simulink model "power_kundur_statcom01"  (R2021a)
settings: Solver=ode23tb  StartTime=0.0  StopTime=10  MaxStep=1/60  RelTol=1e-4  EnableMultiTasking=on
values from neighbouring files (symbols this model uses):
  j = 1    [OABC_PSO_TUNED_NOFault.mat]    (also in OABC_PSO_TUNED_ThreePHASEFault.mat; Traditional_ABC_PSO2.m = randi([1 noFood], 1))
  kk = [0 0.302628193662]    [OABC_PSO_TUNED_NOFault.mat]    (also in OABC_PSO_TUNED_ThreePHASEFault.mat = [6.69502367045 1584.585174])
undefined symbols (not defined in the file or in its folder): Ac, Bc, Cc, D1, Dc, Delta, Fnom, gcbh, K_Vdq2m_SH, Kf_I_SH, Ki_I_SH, Ki_Vac_SH, Ki_Vdc_SH, Kp_I_SH, Kp_Vac_SH, Kp_Vdc_SH, L_RL_SH, MagIinit_SH, PhaIinit_SH, R_RL_SH, sps_rtmsupport, VdcRef_SH, Vnom_SH, xfo_ratio_SH
libraries: spsGenericPowerSystemStabilizerLib x8, spsLoadFlowBusLib x6, spsThreePhaseParallelRLCLoadLib x4, spsThreePhasePISectionLineLib x4, spsSynchronousMachinepuStandardLib x4, spsExcitationSystemLib x4, spsMultiBandPowerSystemStabilizerLib x4, spsSteamTurbineandGovernorLib x4, spsThreePhaseTransformerTwoWindingsLib x4, spsThreePhaseVIMeasurementLib x3, spsThreePhaseBreakerLib x2, spsControlledCurrentSourceLib x2
(part 1 of 3)
Description:
  | Copyright 2008-2015 The MathWorks, Inc.
settings Model: FPTRunName=Active  ExtModeTrigMode=oneshot  ExtModeArmWhenConnect=off  ExtModeAutoUpdateStatusClock=off  Creator=MathWorks  LastModifiedBy=USER
settings SolverCC: AlgebraicLoopSolver=TrustRegion
settings DataIOCC: SaveFormat=Array  SignalLoggingSaveFormat=ModelDataLogs  SaveOutput=off  SaveTime=off  ReturnWorkspaceOutputs=off  TimeSaveName=t  SignalLoggingName=sigsOut
settings OptimizationCC: BlockReduction=off  BooleanDataType=off  ExpressionDepthLimit=2147483647  InitFltsAndDblsToZero=on  LifeSpan=inf
settings DebuggingCC: UnderspecifiedInitializationDetection=Classic  MergeDetectMultiDrivingBlocksExec=none  SignalResolutionControl=TryResolveAllWithWarning  MultiTaskDSMMsg=warning  MultiTaskCondExecSysMsg=none  FcnCallInpInsideContextMsg=warning  UnconnectedOutputMsg=none  StateNameClashWarn=warning  SFUnexpectedBacktrackingDiag=warning  SFNoUnconditionalDefaultTransitionDiag=warning  SFExecutionAtInitializationDiag=none  SFMachineParentedDataDiag=warning  ArithmeticOperatorsInVariantConditions=warning
settings HardwareCC: ProdBitPerPointer=32  ProdBitPerSizeT=32  ProdBitPerPtrDiffT=32  ProdLargestAtomicFloat=None  ProdIntDivRoundTo=Undefined  ProdEndianess=Unspecified  ProdWordSize=32  ProdHWDeviceType=32-bit Generic  TargetUnknown=on
settings ModelReferenceCC: PropagateSignalLabelsOutOfModel=off
settings SFSimCC: SimUseLocalCustomCode=off  CustomCodeUndefinedFunction=UseInterfaceOnly
settings RTWCC: RTWUseLocalCustomCode=off
settings CodeAppCC: StateflowObjectComments=on
settings GRTTargetCC: TargetLangStandard=C89/C90 (ANSI)  CombineOutputUpdateFcns=off  GRTInterface=on
settings ConfigComp: CovMetricSettings=dw  CovSaveCumulativeToWorkspaceVar=on  CovSaveSingleToWorkspaceVar=on  CovExternalEMLEnable=off  CovSFcnEnable=off
settings SimscapeCC: SimscapeNormalizeSystem=off

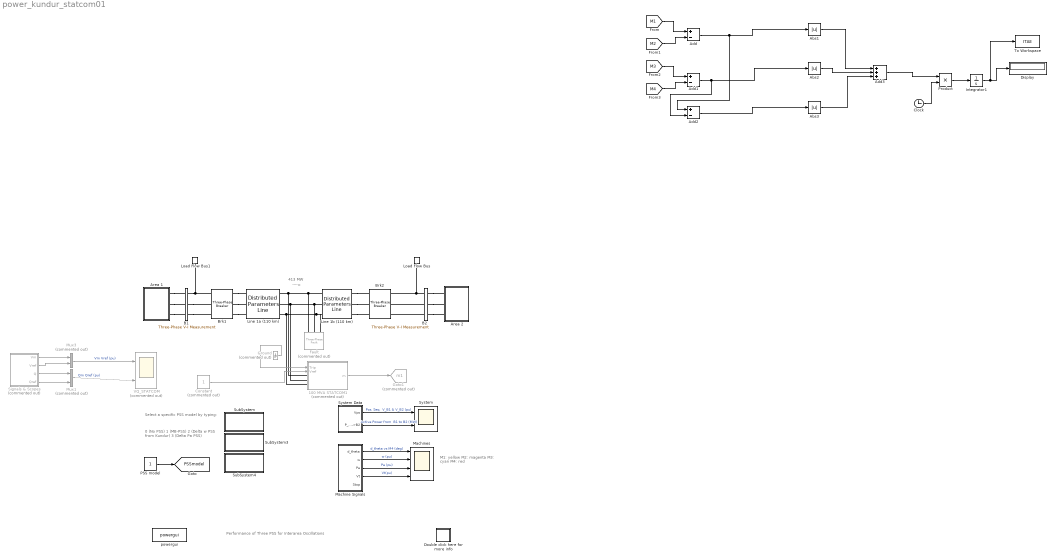
== system power_kundur_statcom01 ==
  note: Performance of Three PSS for Interarea Oscillations
  note: M1: yellow
      | M2: magenta
      | M3: cyan
      | M4: red
  note: ---->
  note: 413 MW
  note: Select a specific PSS model
      | by typing:
  note: 0  (No PSS)
      | 1  (MB-PSS)
      | 2  (Delta w PSS from Kundur)
      | 3  (Delta Pa PSS)
  " Brk2" : spsThreePhaseBreakerLib/Three-Phase Breaker  InitialState=closed  SwitchA=off  SwitchB=off  SwitchC=off  SwitchTimes=[1+8/60]  External=off  BreakerResistance=0.001  SnubberResistance=1e6  SnubberCapacitance=0  Measurements=None
      settings: AttributesFormatString=\n
  100 MVA STATCOM1 : Subsystem  Commented=on  AncestorBlock=|  DialogController=POWERSYS.PowerSysDialog  LoadFcn=sps_rtmsupport('LoadFcn',gcbh);  StartFcn=sps_rtmsupport('StartFcn',gcbh);  StopFcn=sps_rtmsupport('StopFcn',gcbh);  mask(Static Synchronous Compensator (Phasor Type)){SystemNominal=[ 230e3, 60 ], Pnom_SH=200e6, RL_SH=[ 0.071, 0.22 ], Iinit_SH=[0, 0 ], VnomDC=40000, C_DC=750e-6/2, OpMode_SH=Voltage regulation, Vref_SH=1.00, ExternalVref=on, MaxRateChangeVref_SH=100, Droop_SH=0.03, Par_VacReg=[kk(1) kk(2)], Qref_SH=0, MaxRateChangeQref_SH=2, Par_VdcReg=[kk(3) kk(4)], Par_IReg_SH=[0.3 10 0.22]}
      | factslib/Power-Electronics Based
      | FACTS/Static Synchronous
      | Compensator
      | (Phasor Type)
      mask prompts: SystemNominal "Nominal voltage and frequency [Vrms L-L, fn(Hz)]:"; Pnom_SH "Converter rating (VA):"; RL_SH "Converter impedance [R(pu), L(pu)]:"; Iinit_SH "Converter initial current [Mag(pu), Pha(deg.)]:"; VnomDC "DC link nominal voltage (V):"; C_DC "DC link total equivalent capacitance (F):"; OpMode_SH "Mode:"; Vref_SH "Reference voltage Vref (pu):"; ExternalVref "External"; MaxRateChangeVref_SH "Maximum rate of change of reference voltage (pu/s):"; Droop_SH "Droop (pu):"; Par_VacReg "Vac Regulator gains [Kp, Ki]:"; Qref_SH "Reactive power setpoint Qref (pu):"; MaxRateChangeQref_SH "Maximum rate of change of reactive power setpoint (pu/s):"; Par_VdcReg "Vdc Regulator gains [Kp, Ki]:"; Par_IReg_SH "Current Regulator gains [Kp, Ki, Kf];"
      mask help: Implement phasor model of three-phase static synchronous compensator (STATCOM).
      mask init:
      | [ j,Fnom,Vnom_SH,VdcRef_SH,R_RL_SH,L_RL_SH,Kp_Vac_SH,Ki_Vac_SH,Kp_Vdc_SH,Ki_Vdc_SH,Kp_I_SH,Ki_I_SH,Kf_I_SH,VconvMax_pu,VconvMaxPrim,m_max,VconvMaxSec,xfo_ratio_SH,K_Vdq2m_SH,a,a2,MagIinit_SH,PhaIinit_SH] = powericon('StatcomInit',SystemNominal,VnomDC,Par_VacReg, Par_VdcReg, Par_IReg_SH,Iinit_SH,gcbh,RL_SH);
      settings: CopyFcn=sps_rtmsupport('CopyFcn',gcbh);  DeleteFcn=sps_rtmsupport('DeleteFcn',gcbh);  UndoDeleteFcn=sps_rtmsupport('UndoDeleteFcn',gcbh);  ModelCloseFcn=sps_rtmsupport('ModelCloseFcn',gcbh);  PreSaveFcn=sps_rtmsupport('PreSaveFcn',gcbh);  PostSaveFcn=sps_rtmsupport('PostSaveFcn',gcbh);  NameChangeFcn=sps_rtmsupport('NameChangeFcn',gcbh);  PreCopyFcn=sps_rtmsupport('PreCopyFcn',gcbh);  OpenFcn=sps_rtmsupport('OpenFcn',gcbh, [7 9]);  CloseFcn=sps_rtmsupport('CloseFcn',gcbh);  PreDeleteFcn=sps_rtmsupport('PreDeleteFcn',gcbh);
      mask Help: helpview(psbhelp);
      mask TypeOptions OpMode_SH: Var Control | Voltage regulation
      mask Callback OpMode_SH: StatcomCback(gcbh);
      mask Callback ExternalVref: StatcomCback(gcbh);
      mask DialogControl powerdata Prompt: Power
      mask DialogControl control Prompt: Controller
      mask Display:
      | color('blue');
      | disp('STATCOM')
  Abs1 : Abs
  Abs2 : Abs
  Abs3 : Abs
  Add : Sum  Inputs=+-
  Add1 : Sum  Inputs=+-
  Add2 : Sum  Inputs=+-
  Add3 : Sum  Inputs=+++
  Area 1 : Subsystem
  Area 2 : Subsystem
  B1 : spsThreePhaseVIMeasurementLib/Three-Phase V-I Measurement  VoltageMeasurement=phase-to-ground  SetLabelV=on  LabelV=Vabc_B1  Vpu=off  VpuLL=off  CurrentMeasurement=yes  SetLabelI=on  LabelI=Iabc_B1  Ipu=off  Pbase=100e6  Vbase=500e3  OutputType=Complex  PhasorSimulation=on  PSBequivalent=0
  B2 : spsThreePhaseVIMeasurementLib/Three-Phase V-I Measurement  VoltageMeasurement=phase-to-ground  SetLabelV=on  LabelV=Vabc_B2  Vpu=off  VpuLL=off  CurrentMeasurement=yes  SetLabelI=on  LabelI=Iabc_B2  Ipu=off  Pbase=100e6  Vbase=500e3  OutputType=Complex  PhasorSimulation=on  PSBequivalent=0
  Brk1 : spsThreePhaseBreakerLib/Three-Phase Breaker  InitialState=closed  SwitchA=off  SwitchB=off  SwitchC=off  SwitchTimes=[1+8/60]  External=off  BreakerResistance=0.001  SnubberResistance=inf  SnubberCapacitance=0  Measurements=None
      settings: AttributesFormatString=\n
  Clock : Clock
  Constant : Constant  Commented=on
  Display : Display
  Double click here for more info : Subsystem
      settings: OpenFcn=showdemo(bdroot(gcb))
      mask Display: disp('?')
  Fault : spsThreePhaseFaultLib/Three-Phase Fault  Commented=on  InitialStates=0  FaultA=on  FaultB=on  FaultC=on  GroundFault=on  SwitchTimes=[ 1 1+12/60]  External=off  SwitchStatus=NaN  FaultResistance=0.001  GroundResistance=0.001  SnubberResistance=inf  SnubberCapacitance=0  Measurements=Fault voltages and currents
  Goto1 : Goto  Commented=on  GotoTag=m1  TagVisibility=global
  Ground : Ground  Commented=on
  Integrator1 : Integrator
  Line 1a (110 km) : spsDistributedParametersLineLib/Distributed Parameters Line  Phases=3  Length=110  Frequency=60  Resistance=[0.0001*529 1.61]  Inductance=[0.001*529/(377) 0.0061]  Capacitance=[0.00175/529/(377) 5.2489e-9]  x1=[1.07105753768753e-08 249286.617062631 249286.103987125;376.991118430775 376.991118430775 376.991118430775;-0.430181636815253 0.685365733894338 -0.885427065915489]  x2=[1.12823805694267e-08 223892.22603189 223891.788922386;376.991118430775 376.991118430775 376.991118430775;-0.654447081019999 0.431460957299027 -1.13933225811238]  x3=[6.57239902882849e-12 568.631458690706 568.631298110426;376.991118430775 376.991118430775 376.991118430775;-1.56783526225894 3.01615797225432 1.44536743576562]  x4=[1.40882222020251e-11 1660.67806578935 1660.67616695075;376.991118430775 376.991118430775 376.991118430775;-0.32396524232274 0.29261475856702 -1.27817771618835]  x5=0.000622431770558027  V1=ones(3,3)  V2=ones(3,3)  I1=ones(3,3)  I2=ones(3,3)  nHarmo=1  Measurements=None  Decoupling=off  VsMag0=0  VrMag0=0  VsAngle0=0  VrAngle0=0  IsMag0=0  IrMag0=0  IsAngle0=0  IrAngle0=0
      settings: AttributesFormatString=\n  SourceProductBaseCode=PS
  Line 1b (110 km) : spsDistributedParametersLineLib/Distributed Parameters Line  Phases=3  Length=110  Frequency=60  Resistance=[0.0001*529 1.61]  Inductance=[0.001*529/(377) 0.0061]  Capacitance=[0.00175/529/(377) 5.2489e-9]  x1=[1.12823805694267e-08 223892.22603189 223891.788922386;376.991118430775 376.991118430775 376.991118430775;-0.654447081019999 0.431460957299027 -1.13933225811238]  x2=[1.2011449678639e-08 211111.793515844 211111.458207578;376.991118430775 376.991118430775 376.991118430775;-0.792576364184504 0.132665789252052 -1.4381277782236]  x3=[8.25606215961616e-12 584.178043584259 584.177876576689;376.991118430775 376.991118430775 376.991118430775;-1.38577443880165 -3.11450148556165 1.59789324135678]  x4=[1.24190041898095e-11 1644.49352968555 1644.49164426305;376.991118430775 376.991118430775 376.991118430775;-0.543069260432015 0.147593243960904 -1.42319923514757]  x5=0.000622431770558027  V1=ones(3,3)  V2=ones(3,3)  I1=ones(3,3)  I2=ones(3,3)  nHarmo=1  Measurements=None  Decoupling=off  VsMag0=0  VrMag0=0  VsAngle0=0  VrAngle0=0  IsMag0=0  IrMag0=0  IsAngle0=0  IrAngle0=0
      settings: AttributesFormatString=\n  SourceProductBaseCode=PS
  Load Flow Bus : spsLoadFlowBusLib/Load Flow Bus  LConnTagsString=a  Phases=single  Connectors=on one side  ID=B2  Vbase=230e3  Vref=1  Vangle=0  VLF=1.003  VLFb=1  VLFc=1  angleLF=-11.43  angleLFb=0  angleLFc=0
      settings: AttributesFormatString=%<ID>\n%<Vbase>V\n%<VLF>pu\n%<angleLF>deg.  SourceProductBaseCode=PS
  Load Flow Bus1 : spsLoadFlowBusLib/Load Flow Bus  LConnTagsString=a  Phases=single  Connectors=on one side  ID=B1  Vbase=230e3  Vref=1  Vangle=0  VLF=0.9916  VLFb=1  VLFc=1  angleLF=15.06  angleLFb=0  angleLFc=0
      settings: AttributesFormatString=%<ID>\n%<Vbase>V\n%<VLF>pu\n%<angleLF>deg.  SourceProductBaseCode=PS
  Machine Signals : Subsystem
  Machines : Scope  NumInputPorts=4
  Mux1 : Mux  Commented=on  Inputs=2
  Mux3 : Mux  Commented=on  Inputs=2
  PSS model : Constant
  Product : Product
  Signals & Scopes : Subsystem  Commented=on
  SubSystem : Subsystem
      settings: OpenFcn=openfig('psbPSSbode.fig');
      mask Display: disp('Show Bode plot \nof PSS')
  SubSystem3 : Subsystem
      settings: OpenFcn=openfig('psbPSSstep.fig');
      mask Display: disp('Show results: \nStep on vref\nof M1')
  SubSystem4 : Subsystem
      settings: OpenFcn=openfig('psbPSSfault.fig');
      mask Display: disp('Show results: \n3-phase fault')
  System : Scope  NumInputPorts=2
  System Data : Subsystem
  To Workspace : ToWorkspace  VariableName=ITAE  SampleTime=-1
      settings: Save2DSignal=2-D array (concatenate along first dimension)
  VQ_STATCOM : Scope  Commented=on  NumInputPorts=2
  powergui : spspowerguiLib/powergui  Priority=2  SimulationMode=Phasor  SampleTime=0  frequency=60  Iterations=50  frequencyindice=60  Pbase=100e6  ErrMax=0.0001  UnitsV=kV  UnitsW=MW  buscounter=0  FunctionMessages=off  echomessages=on  EnableUseOfTLC=off  CurrentSourceSwitches=off  DisableSnubberDevices=off  DisableRonSwitches=off  DisableVfSwitches=off  DisplayEquations=off  AutomaticDiscreteSolvers=off  SolverType=Tustin  Interpol=off  ExternalGateDelay=off  methode=off  Ts=0  x0status=blocks  SPID=off  SwTol=0  HookPort=off  NonlinearTolerance=1e-4  nMaxIteration=100  ContinueOnMaxIteration=off  RestoreLinks=warning  ResistiveCurrentMeasurement=off  Frange=logspace(0,3,50)  Ylog=off  Xlog=off  ShowGrid=off  save=off  variable=ZData  structure=0  ZoomFFT=on  StartTime=0.0  cycles=1  DisplayStyle=1  fundamental=60  FreqAxis=off  MaxFrequency=1000  frequencyindicesteady=1  RmsSteady=1  display=off
  tag scope: PSSmodel=global
  wires:
  Machine Signals/1(d_theta) -> Machines/1  "d_theta vs M4 (deg)"
  Machine Signals/2(w) -> Machines/2  "w (pu)"
  Machine Signals/3(Pa) -> Machines/3  "Pa (pu)"
  Machine Signals/4(Vt) -> Machines/4  "Vt(pu)"
  System Data/1(Vps) -> System/1  "Pos. Seq.  V_B1 & V_B2 (pu)"
  System Data/2(P_B1->B2) -> System/2  "Active Power from  B1 to B2 (MW)"
  PSS model/1 -> [PSSmodel]
  Constant/1 -> 100 MVA STATCOM1/2("Vref ")
  Ground/1 -> 100 MVA STATCOM1/1(Trip)
  Signals & Scopes/1(Vm) -> Mux3/1
  Signals & Scopes/2(Vref) -> Mux3/2
  Signals & Scopes/3(Q) -> Mux1/1
  Signals & Scopes/4(Qref) -> Mux1/2
  Mux3/1 -> VQ_STATCOM/1  "Vm Vref (pu)"
  Mux1/1 -> VQ_STATCOM/2  "Qm Qref (pu)"
  100 MVA STATCOM1/1(m) -> Goto1/1
  Clock/1 -> Product/2
  Product/1 -> Integrator1/1
  Integrator1/1 -> To Workspace/1, Display/1
  [M1] -> Add/1
  [M2] -> Add/2
  Add/1 -> Add2/1, Abs1/1
  Add1/1 -> Add2/2, Abs2/1
  [M3] -> Add1/1
  [M4] -> Add1/2
  Add2/1 -> Abs3/1
  Abs1/1 -> Add3/1
  Abs2/1 -> Add3/2
  Abs3/1 -> Add3/3
  Add3/1 -> Product/1
  connections:
  Brk1/RConn1 -- Line 1a (110 km)/LConn1
  Brk1/RConn2 -- Line 1a (110 km)/LConn2
  Brk1/RConn3 -- Line 1a (110 km)/LConn3
  Line 1b (110 km)/LConn1 -- 100 MVA STATCOM1/LConn1 -- Line 1a (110 km)/RConn1 -- Fault/LConn1
  Line 1b (110 km)/LConn2 -- 100 MVA STATCOM1/LConn2 -- Line 1a (110 km)/RConn2 -- Fault/LConn2
  Line 1a (110 km)/RConn3 -- Line 1b (110 km)/LConn3 -- Fault/LConn3 -- 100 MVA STATCOM1/LConn3
  Line 1b (110 km)/RConn1 -- " Brk2"/LConn1
  Line 1b (110 km)/RConn2 -- " Brk2"/LConn2
  Line 1b (110 km)/RConn3 -- " Brk2"/LConn3
  Area 1/RConn2 -- B1/LConn2
  Area 1/RConn1 -- B1/LConn1
  Area 1/RConn3 -- B1/LConn3
  B1/RConn2 -- Brk1/LConn2
  B1/RConn1 -- Brk1/LConn1 -- Load Flow Bus1/LConn1
  B1/RConn3 -- Brk1/LConn3
  B2/RConn2 -- Area 2/LConn2
  B2/RConn1 -- Area 2/LConn1
  B2/RConn3 -- Area 2/LConn3
  B2/LConn2 -- " Brk2"/RConn2
  B2/LConn1 -- " Brk2"/RConn1 -- Load Flow Bus/LConn1
  B2/LConn3 -- " Brk2"/RConn3

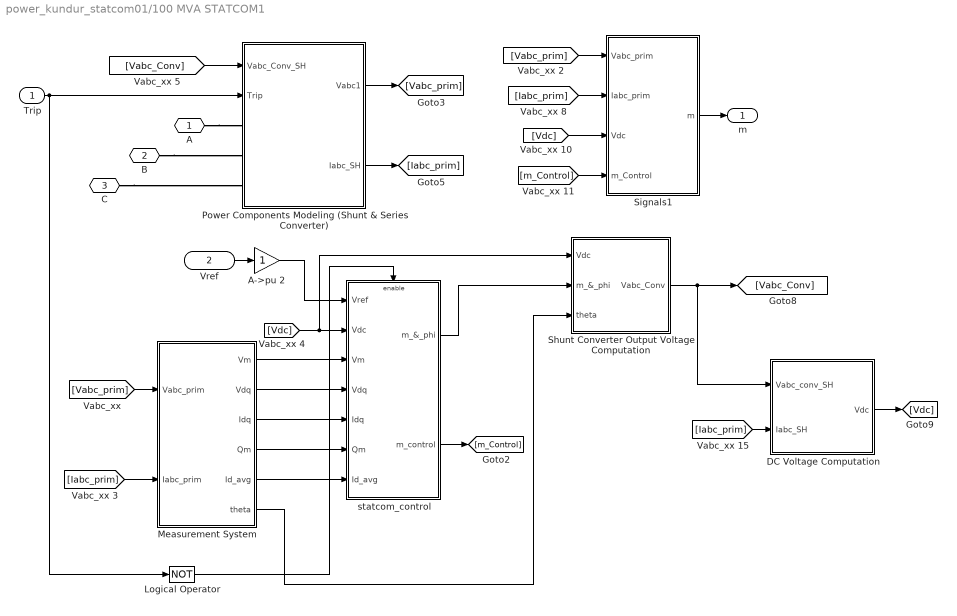
== system power_kundur_statcom01/100 MVA STATCOM1 ==
  Trip : Inport
  "Vref " : Inport  Port=2
  A->pu 2 : Gain  SaturateOnIntegerOverflow=on  SampleTime=0  OutDataTypeStr=Inherit: Same as input  ParamDataTypeStr=Inherit: Same as input
  DC Voltage Computation : Subsystem
  Logical Operator : Logic  Operator=NOT  AllPortsSameDT=off  OutDataTypeStr=float('double')  SampleTime=0
  Measurement System : Subsystem  mask{Vm_SH_Init=1, Id_avg_SH_Init=0, Qm_SH_Init=0, Fnom=Fnom, Vnom_SH=Vnom_SH, Pnom_SH=Pnom_SH}
      mask prompts: Vm_SH_Init "Initial value for Vm_SH (pu):"; Id_avg_SH_Init "Initial value for Id_avg_SH (pu):"; Qm_SH_Init "Initial value for Qm_SH (pu):"; Fnom "System frequency (Hz):"
  Power Components Modeling (Shunt & Series Converter) : Subsystem
  Shunt Converter Output Voltage Computation : Subsystem
  Signals1 : Subsystem
  statcom_control : Subsystem
  "A " : PMIOPort  Side=Left
  B : PMIOPort  Port=2  Side=Left
  C : PMIOPort  Port=3  Side=Left
  m : Outport  VectorParamsAs1DForOutWhenUnconnected=off
  wires:
  statcom_control/2(m_control) -> [m_Control]
  Logical Operator/1 -> statcom_control/Enable
  Measurement System/5(Id_avg) -> statcom_control/7(Id_avg)
  Measurement System/4(Qm) -> statcom_control/6(Qm)
  Trip/1 -> Logical Operator/1, Power Components Modeling (Shunt & Series Converter)/2(Trip)
  Measurement System/6(theta) -> Shunt Converter Output Voltage Computation/3(theta)
  [Vdc] -> statcom_control/2(Vdc), Shunt Converter Output Voltage Computation/1(Vdc)
  A->pu 2/1 -> statcom_control/1(Vref)
  [Vabc_prim] -> Measurement System/1(Vabc_prim)
  [Iabc_prim] -> Measurement System/2(Iabc_prim)
  Measurement System/3(Idq) -> statcom_control/5(Idq)
  Measurement System/2(Vdq) -> statcom_control/4(Vdq)
  Measurement System/1(Vm) -> statcom_control/3(Vm)
  DC Voltage Computation/1(Vdc) -> [Vdc]
  [Iabc_prim] -> DC Voltage Computation/2(Iabc_SH)
  Shunt Converter Output Voltage Computation/1(Vabc_Conv) -> DC Voltage Computation/1(Vabc_conv_SH), [Vabc_Conv]
  [m_Control] -> Signals1/4(m_Control)
  [Vdc] -> Signals1/3(Vdc)
  [Iabc_prim] -> Signals1/2(Iabc_prim)
  [Vabc_prim] -> Signals1/1(Vabc_prim)
  Power Components Modeling (Shunt & Series Converter)/2(Iabc_SH) -> [Iabc_prim]
  Power Components Modeling (Shunt & Series Converter)/1(Vabc1) -> [Vabc_prim]
  [Vabc_Conv] -> Power Components Modeling (Shunt & Series Converter)/1(Vabc_Conv_SH)
  Signals1/1(m) -> m/1
  statcom_control/1(m_&_phi) -> Shunt Converter Output Voltage Computation/2(m_&_phi)
  "Vref "/1 -> A->pu 2/1
  connections:
  C/RConn1 -- Power Components Modeling (Shunt & Series Converter)/LConn3
  B/RConn1 -- Power Components Modeling (Shunt & Series Converter)/LConn2
  "A "/RConn1 -- Power Components Modeling (Shunt & Series Converter)/LConn1

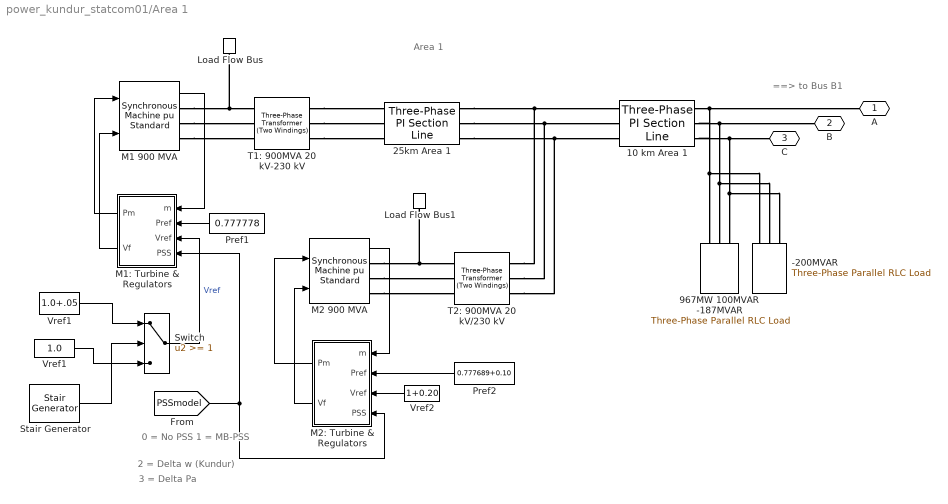
== system power_kundur_statcom01/Area 1 ==
  note: Area 1
  note: ==> to Bus B1
  note: 0 = No PSS
      | 1 = MB-PSS
  note: 3 = Delta Pa
  note: 2 = Delta w (Kundur)
  -200MVAR : spsThreePhaseParallelRLCLoadLib/Three-Phase Parallel RLC Load  LConnTagsString=A|B|C  Configuration=Y (grounded)  NominalVoltage=230e3  Vabc=[1e3 1e3 1e3]  Vabcp=[1e3 1e3 1e3]  NominalFrequency=60  UnbalancedPower=off  ActivePower=0  InductivePower=0  CapacitivePower=200e6  Pabc=[10e3 9e3 11e3]  QLabc=[100 90 110]  QCabc=[100 90 110]  Pabcp=[10e3 9e3 11e3]  QLabcp=[100 90 110]  QCabcp=[100 90 110]  Measurements=None  LoadType=constant Z
  10 km Area 1 : spsThreePhasePISectionLineLib/Three-Phase PI Section Line  LConnTagsString=a|b|c  RConnTagsString=A|B|C  Length=10  Frequency=60  Resistances=[0.0001*529 1.61]  Inductances=[0.001*529/(377) 0.0061]  Capacitances=[0.00175/529/(377) 5.2489e-9]
  25km Area 1 : spsThreePhasePISectionLineLib/Three-Phase PI Section Line  LConnTagsString=a|b|c  RConnTagsString=A|B|C  Length=25  Frequency=60  Resistances=[0.0001*529 1.61]  Inductances=[0.001*529/(377) 0.0061]  Capacitances=[0.00175/529/(377) 5.2489e-9]
  967MW 100MVAR -187MVAR : spsThreePhaseParallelRLCLoadLib/Three-Phase Parallel RLC Load  LConnTagsString=A|B|C  Configuration=Y (grounded)  NominalVoltage=230e3  Vabc=[1e3 1e3 1e3]  Vabcp=[1e3 1e3 1e3]  NominalFrequency=60  UnbalancedPower=off  ActivePower=967000000+96700000  InductivePower=100e6  CapacitivePower=187e6  Pabc=[10e3 9e3 11e3]  QLabc=[100 90 110]  QCabc=[100 90 110]  Pabcp=[10e3 9e3 11e3]  QLabcp=[100 90 110]  QCabcp=[100 90 110]  Measurements=None  LoadType=constant Z
  Load Flow Bus : spsLoadFlowBusLib/Load Flow Bus  LConnTagsString=a  Phases=single  Connectors=on one side  ID=M1_Area1  Vbase=20e3  Vref=1  Vangle=0  VLF=1  VLFb=1  VLFc=1  angleLF=10.22  angleLFb=0  angleLFc=0
      settings: AttributesFormatString=%<ID>\n%<Vbase>V\n%<VLF>pu\n%<angleLF>deg.  SourceProductBaseCode=PS
  Load Flow Bus1 : spsLoadFlowBusLib/Load Flow Bus  LConnTagsString=a  Phases=single  Connectors=on one side  ID=M2_Area1  Vbase=20e3  Vref=1  Vangle=0  VLF=1  VLFb=1  VLFc=1  angleLF=0  angleLFb=0  angleLFc=0
      settings: AttributesFormatString=%<ID>\n%<Vbase>V\n%<VLF>pu\n%<angleLF>deg.  SourceProductBaseCode=PS
  M1 900 MVA : spsSynchronousMachinepuStandardLib/Synchronous Machine pu Standard  PresetModel=No  MechanicalLoad=Mechanical power Pm  ShowDetailedParameters=on  RotorType=Round  Units=per unit standard parameters  MeasurementBus=off  NominalParameters="[900E6  20000   60 ]"  Reactances1=[1.8 .3 .25 1.7 .55 .25 .2]  Reactances2=[ 1.305, 0.296, 0.252, 0.474, 0.243, 0.18 ]  dAxisTimeConstants=Open-circuit  qAxisTimeConstants=Open-circuit  TimeConstants1=[]  TimeConstants2=[8 .03 .4 .05]  TimeConstants3=[]  TimeConstants4=[]  TimeConstants5=[ 1.01, 0.053, 0.1 ]  TimeConstants6=[]  TimeConstants7=[]  TimeConstants8=[]  StatorResistance=0.0025  Mechanical=[ 6.5 0 4]  PolePairs=4  InitialConditions=[0 -31.4247 0.784453 0.784453 0.784453 2.7401 -117.26 122.74 1.83395]  SetSaturation=off  Saturation=[0.6404,0.7127,0.8441,0.9214,0.9956,1.082,1.19,1.316,1.457;0.7,0.7698,0.8872,0.9466,0.9969,1.046,1.1,1.151,1.201]  LoadFlowParameters=[1 700000000 0 0 0]  TsPowergui=0  TsBlock=-1  IterativeModel=Trapezoidal non iterative  IterativeDiscreteModel=Trapezoidal non iterative  BusType=PV  Pref=700000000  Qref=0  Qmin=-Inf  Qmax=Inf  PLF=0  QLF=0
      settings: SourceProductBaseCode=PS
  M1: Turbine & Regulators : Subsystem
  M2 900 MVA : spsSynchronousMachinepuStandardLib/Synchronous Machine pu Standard  PresetModel=No  MechanicalLoad=Mechanical power Pm  ShowDetailedParameters=on  RotorType=Round  Units=per unit standard parameters  MeasurementBus=off  NominalParameters="[900E6  20000   60 ]"  Reactances1=[1.8 .3 .25 1.7 .55 .25 .2]  Reactances2=[ 1.305, 0.296, 0.252, 0.474, 0.243, 0.18 ]  dAxisTimeConstants=Open-circuit  qAxisTimeConstants=Open-circuit  TimeConstants1=[]  TimeConstants2=[8 .03 .4 .05]  TimeConstants3=[]  TimeConstants4=[]  TimeConstants5=[ 1.01, 0.053, 0.1 ]  TimeConstants6=[]  TimeConstants7=[]  TimeConstants8=[]  StatorResistance=0.0025  Mechanical=[ 6.5 0 4]  PolePairs=4  InitialConditions=[0 -42.8075 0.788608 0.788608 0.788608 -9.54571 -129.546 110.454 1.86756]  SetSaturation=off  Saturation=[0.6404,0.7127,0.8441,0.9214,0.9956,1.082,1.19,1.316,1.457;0.7,0.7698,0.8872,0.9466,0.9969,1.046,1.1,1.151,1.201]  LoadFlowParameters=[2 700000000 0 0 0]  TsPowergui=0  TsBlock=-1  IterativeModel=Trapezoidal non iterative  IterativeDiscreteModel=Trapezoidal non iterative  BusType=swing  Pref=0  Qref=0  Qmin=-Inf  Qmax=Inf  PLF=0  QLF=0
      settings: SourceProductBaseCode=PS
  M2: Turbine & Regulators : Subsystem
  Pref1 : Constant  Value=0.777778
  Pref2 : Constant  Value=0.777689+0.10
  Stair Generator : spsStairGeneratorLib/Stair Generator  t=[0 1 1.2]*100  e=[0 1 0 ]  Ts=0
  Switch : Switch  Threshold=1  InputSameDT=on
  T1: 900MVA 20 kV-230 kV : spsThreePhaseTransformerTwoWindingsLib/Three-Phase Transformer (Two Windings)  Winding1Connection=Delta (D1)  Winding2Connection=Yg  CoreType=Three single-phase transformers  SetSaturation=off  Hysteresis=off  DataFile='hysteresis'  SetInitialFlux=off  Measurements=None  UNITS=pu  NominalPower="[ 900e6   60 ]"  Winding1="[ 20e3  1e-6   0  ]"  Winding2="[ 230e3  1e-6   0.15 ]"  Rm=500  Lm=500  L0=0.5  Saturation="[ 0,0  ;  0.005,1.2  ;  1.0,1.4 ]"  InitialFluxes=[ 0.8 , -0.8 , 0.7 ]  BreakLoop=off  DiscreteSolver=Trapezoidal iterative  DataType=off  TransfoNumber=0
  T2: 900MVA 20 kV/230 kV : spsThreePhaseTransformerTwoWindingsLib/Three-Phase Transformer (Two Windings)  Winding1Connection=Delta (D1)  Winding2Connection=Yg  CoreType=Three single-phase transformers  SetSaturation=off  Hysteresis=off  DataFile='hysteresis'  SetInitialFlux=off  Measurements=None  UNITS=pu  NominalPower=[ 900e6 60 ]  Winding1="[ 20e3 1e-6  0.0]"  Winding2=[ 230e3 1e-6 0.15]  Rm=500  Lm=500  L0=0.5  Saturation="[ 0,0  ;  0.005,1.2  ;  1.0,1.4 ]"  InitialFluxes=[ 0.8 , -0.8 , 0.7 ]  BreakLoop=off  DiscreteSolver=Trapezoidal iterative  DataType=off  TransfoNumber=0
  Vref1 : Constant  Value=1.0
  "Vref1 " : Constant  Value=1.0+.05
  Vref2 : Constant  Value=1+0.20
  " A" : PMIOPort  Side=Right
  " B" : PMIOPort  Port=2  Side=Right
  " C" : PMIOPort  Port=3  Side=Right
  wires:
  Pref1/1 -> M1: Turbine & Regulators/2(Pref)
  Switch/1 -> M1: Turbine & Regulators/3(Vref)  "Vref"
  Stair Generator/1 -> Switch/2
  [PSSmodel] -> M1: Turbine & Regulators/4(PSS), M2: Turbine & Regulators/4(PSS)
  Pref2/1 -> M2: Turbine & Regulators/2(Pref)
  Vref2/1 -> M2: Turbine & Regulators/3(Vref)
  Vref1/1 -> Switch/3
  "Vref1 "/1 -> Switch/1
  M2 900 MVA/1 -> M2: Turbine & Regulators/1(m)
  M2: Turbine & Regulators/1(Pm) -> M2 900 MVA/1
  M2: Turbine & Regulators/2(Vf) -> M2 900 MVA/2
  M1: Turbine & Regulators/1(Pm) -> M1 900 MVA/1
  M1: Turbine & Regulators/2(Vf) -> M1 900 MVA/2
  M1 900 MVA/1 -> M1: Turbine & Regulators/1(m)
  connections:
  T1: 900MVA 20 kV-230 kV/RConn1 -- 25km Area 1/LConn1
  T1: 900MVA 20 kV-230 kV/RConn2 -- 25km Area 1/LConn2
  M2 900 MVA/RConn1 -- T2: 900MVA 20 kV/230 kV/LConn1 -- Load Flow Bus1/LConn1
  M2 900 MVA/RConn2 -- T2: 900MVA 20 kV/230 kV/LConn2
  M2 900 MVA/RConn3 -- T2: 900MVA 20 kV/230 kV/LConn3
  T1: 900MVA 20 kV-230 kV/RConn3 -- 25km Area 1/LConn3
  10 km Area 1/RConn1 -- " A"/RConn1 -- 967MW 100MVAR -187MVAR/LConn1 -- -200MVAR/LConn1
  10 km Area 1/RConn2 -- " B"/RConn1 -- 967MW 100MVAR -187MVAR/LConn2 -- -200MVAR/LConn2
  10 km Area 1/RConn3 -- " C"/RConn1 -- 967MW 100MVAR -187MVAR/LConn3 -- -200MVAR/LConn3
  M1 900 MVA/RConn1 -- T1: 900MVA 20 kV-230 kV/LConn1 -- Load Flow Bus/LConn1
  M1 900 MVA/RConn2 -- T1: 900MVA 20 kV-230 kV/LConn2
  M1 900 MVA/RConn3 -- T1: 900MVA 20 kV-230 kV/LConn3
  25km Area 1/RConn2 -- 10 km Area 1/LConn2 -- T2: 900MVA 20 kV/230 kV/RConn2
  25km Area 1/RConn1 -- 10 km Area 1/LConn1 -- T2: 900MVA 20 kV/230 kV/RConn1
  25km Area 1/RConn3 -- 10 km Area 1/LConn3 -- T2: 900MVA 20 kV/230 kV/RConn3

== system power_kundur_statcom01/Area 2 ==
  note: 2 = Delta w (Kundur)
  note: 3 = Delta Pa
  note: 0 = No PSS
      | 1 = MB-PSS
  note: ==> to Bus B2
  note: Area 2
  -350MVAR : spsThreePhaseParallelRLCLoadLib/Three-Phase Parallel RLC Load  LConnTagsString=A|B|C  Configuration=Y (grounded)  NominalVoltage=230e3  Vabc=[1e3 1e3 1e3]  Vabcp=[1e3 1e3 1e3]  NominalFrequency=60  UnbalancedPower=off  ActivePower=0  InductivePower=0  CapacitivePower=350e6  Pabc=[10e3 9e3 11e3]  QLabc=[100 90 110]  QCabc=[100 90 110]  Pabcp=[10e3 9e3 11e3]  QLabcp=[100 90 110]  QCabcp=[100 90 110]  Measurements=None  LoadType=constant Z
  10 km Area 2 : spsThreePhasePISectionLineLib/Three-Phase PI Section Line  LConnTagsString=a|b|c  RConnTagsString=A|B|C  Length=10  Frequency=60  Resistances=[0.0001*529 1.61]  Inductances=[0.001*529/(377) 0.0061]  Capacitances=[0.00175/529/(377) 5.2489e-9]
  1767MW 100MVAR -187MVAR : spsThreePhaseParallelRLCLoadLib/Three-Phase Parallel RLC Load  LConnTagsString=A|B|C  Configuration=Y (grounded)  NominalVoltage=230e3  Vabc=[1e3 1e3 1e3]  Vabcp=[1e3 1e3 1e3]  NominalFrequency=60  UnbalancedPower=off  ActivePower=1767000000  InductivePower=100e6  CapacitivePower=187e6  Pabc=[10e3 9e3 11e3]  QLabc=[100 90 110]  QCabc=[100 90 110]  Pabcp=[10e3 9e3 11e3]  QLabcp=[100 90 110]  QCabcp=[100 90 110]  Measurements=None  LoadType=constant Z
  25km Area 2 : spsThreePhasePISectionLineLib/Three-Phase PI Section Line  LConnTagsString=a|b|c  RConnTagsString=A|B|C  Length=25  Frequency=60  Resistances=[0.0001*529 1.61]  Inductances=[0.001*529/(377) 0.0061]  Capacitances=[0.00175/529/(377) 5.2489e-9]
  Load Flow Bus : spsLoadFlowBusLib/Load Flow Bus  LConnTagsString=a  Phases=single  Connectors=on one side  ID=M3_Area2  Vbase=20e3  Vref=1  Vangle=0  VLF=1  VLFb=1  VLFc=1  angleLF=-15.88  angleLFb=0  angleLFc=0
      settings: AttributesFormatString=%<ID>\n%<Vbase>V\n%<VLF>pu\n%<angleLF>deg.  SourceProductBaseCode=PS
  Load Flow Bus1 : spsLoadFlowBusLib/Load Flow Bus  LConnTagsString=a  Phases=single  Connectors=on one side  ID=M4_Area2  Vbase=20e3  Vref=1  Vangle=0  VLF=1  VLFb=1  VLFc=1  angleLF=-26.53  angleLFb=0  angleLFc=0
      settings: AttributesFormatString=%<ID>\n%<Vbase>V\n%<VLF>pu\n%<angleLF>deg.  SourceProductBaseCode=PS
  M3 900 MVA : spsSynchronousMachinepuStandardLib/Synchronous Machine pu Standard  PresetModel=No  MechanicalLoad=Mechanical power Pm  ShowDetailedParameters=on  RotorType=Round  Units=per unit standard parameters  MeasurementBus=off  NominalParameters="[900E6  20000   60 ]"  Reactances1=[1.8 .3 .25 1.7 .55 .25 .2]  Reactances2=[ 1.305, 0.296, 0.252, 0.474, 0.243, 0.18 ]  dAxisTimeConstants=Open-circuit  qAxisTimeConstants=Open-circuit  TimeConstants1=[]  TimeConstants2=[8 .03 .4 .05]  TimeConstants3=[]  TimeConstants4=[]  TimeConstants5=[ 1.01, 0.053, 0.1 ]  TimeConstants6=[]  TimeConstants7=[]  TimeConstants8=[]  StatorResistance=0.0025  Mechanical=[ 6.175 0 4]  PolePairs=4  InitialConditions=[0 -56.3243 0.8041 0.8041 0.8041 -22.4087 -142.409 97.5913 1.85092]  SetSaturation=off  Saturation=[0.6404,0.7127,0.8441,0.9214,0.9956,1.082,1.19,1.316,1.457;0.7,0.7698,0.8872,0.9466,0.9969,1.046,1.1,1.151,1.201]  LoadFlowParameters=[1 719000000 0 0 0]  TsPowergui=0  TsBlock=-1  IterativeModel=Trapezoidal non iterative  IterativeDiscreteModel=Trapezoidal non iterative  BusType=PV  Pref=719000000  Qref=0  Qmin=-Inf  Qmax=Inf  PLF=0  QLF=0
      settings: SourceProductBaseCode=PS
  M3: Turbine & Regulators : Subsystem
  M4 900 MVA : spsSynchronousMachinepuStandardLib/Synchronous Machine pu Standard  PresetModel=No  MechanicalLoad=Mechanical power Pm  ShowDetailedParameters=on  RotorType=Round  Units=per unit standard parameters  MeasurementBus=off  NominalParameters="[900E6  20000   60 ]"  Reactances1=[1.8 .3 .25 1.7 .55 .25 .2]  Reactances2=[ 1.305, 0.296, 0.252, 0.474, 0.243, 0.18 ]  dAxisTimeConstants=Open-circuit  qAxisTimeConstants=Open-circuit  TimeConstants1=[]  TimeConstants2=[8 .03 .4 .05]  TimeConstants3=[]  TimeConstants4=[]  TimeConstants5=[ 1.01, 0.053, 0.1 ]  TimeConstants6=[]  TimeConstants7=[]  TimeConstants8=[]  StatorResistance=0.0025  Mechanical=[ 6.175 0 4]  PolePairs=4  InitialConditions=[0 -67.7513 0.783185 0.783185 0.783185 -33.268 -153.268 86.732 1.82209]  SetSaturation=off  Saturation=[0.6404,0.7127,0.8441,0.9214,0.9956,1.082,1.19,1.316,1.457;0.7,0.7698,0.8872,0.9466,0.9969,1.046,1.1,1.151,1.201]  LoadFlowParameters=[1 700000000 0 0 0]  TsPowergui=0  TsBlock=-1  IterativeModel=Trapezoidal non iterative  IterativeDiscreteModel=Trapezoidal non iterative  BusType=PV  Pref=700000000  Qref=0  Qmin=-Inf  Qmax=Inf  PLF=0  QLF=0
      settings: SourceProductBaseCode=PS
  M4: Turbine & Regulators : Subsystem
  Pref3 : Constant  Value=0.798889
  Pref4 : Constant  Value=0.777778
  T3: 900MVA 20 kV-230 kV : spsThreePhaseTransformerTwoWindingsLib/Three-Phase Transformer (Two Windings)  Winding1Connection=Delta (D1)  Winding2Connection=Yg  CoreType=Three single-phase transformers  SetSaturation=off  Hysteresis=off  DataFile='hysteresis'  SetInitialFlux=off  Measurements=None  UNITS=pu  NominalPower="[ 900e6   60 ]"  Winding1="[ 20e3  1e-6   0  ]"  Winding2="[ 230e3  1e-6   0.15 ]"  Rm=500  Lm=500  L0=0.5  Saturation="[ 0,0  ;  0.005,1.2  ;  1.0,1.4 ]"  InitialFluxes=[ 0.8 , -0.8 , 0.7 ]  BreakLoop=off  DiscreteSolver=Trapezoidal iterative  DataType=off  TransfoNumber=0
  T4: 900MVA 20 kV/230 kV : spsThreePhaseTransformerTwoWindingsLib/Three-Phase Transformer (Two Windings)  Winding1Connection=Delta (D1)  Winding2Connection=Yg  CoreType=Three single-phase transformers  SetSaturation=off  Hysteresis=off  DataFile='hysteresis'  SetInitialFlux=off  Measurements=None  UNITS=pu  NominalPower=[ 900e6 60 ]  Winding1="[ 20e3 1e-6  0.0]"  Winding2=[ 230e3 1e-6 0.15]  Rm=500  Lm=500  L0=0.5  Saturation="[ 0,0  ;  0.005,1.2  ;  1.0,1.4 ]"  InitialFluxes=[ 0.8 , -0.8 , 0.7 ]  BreakLoop=off  DiscreteSolver=Trapezoidal iterative  DataType=off  TransfoNumber=0
  Vref3 : Constant  Value=1.0
  Vref4 : Constant
  A : PMIOPort  Side=Left
  B : PMIOPort  Port=2  Side=Left
  C : PMIOPort  Port=3  Side=Left
  wires:
  [PSSmodel] -> M3: Turbine & Regulators/4(PSS), M4: Turbine & Regulators/4(PSS)
  Pref3/1 -> M3: Turbine & Regulators/2(Pref)
  Vref3/1 -> M3: Turbine & Regulators/3(Vref)
  Pref4/1 -> M4: Turbine & Regulators/2(Pref)
  Vref4/1 -> M4: Turbine & Regulators/3(Vref)
  M3 900 MVA/1 -> M3: Turbine & Regulators/1(m)
  M3: Turbine & Regulators/2(Vf) -> M3 900 MVA/2
  M3: Turbine & Regulators/1(Pm) -> M3 900 MVA/1
  M4: Turbine & Regulators/1(Pm) -> M4 900 MVA/1
  M4: Turbine & Regulators/2(Vf) -> M4 900 MVA/2
  M4 900 MVA/1 -> M4: Turbine & Regulators/1(m)
  connections:
  M3 900 MVA/RConn3 -- T3: 900MVA 20 kV-230 kV/LConn3
  M3 900 MVA/RConn2 -- T3: 900MVA 20 kV-230 kV/LConn2
  M3 900 MVA/RConn1 -- T3: 900MVA 20 kV-230 kV/LConn1 -- Load Flow Bus/LConn1
  T3: 900MVA 20 kV-230 kV/RConn3 -- 25km Area 2/LConn3
  M4 900 MVA/RConn3 -- T4: 900MVA 20 kV/230 kV/LConn3
  M4 900 MVA/RConn2 -- T4: 900MVA 20 kV/230 kV/LConn2
  M4 900 MVA/RConn1 -- T4: 900MVA 20 kV/230 kV/LConn1 -- Load Flow Bus1/LConn1
  T3: 900MVA 20 kV-230 kV/RConn2 -- 25km Area 2/LConn2
  T3: 900MVA 20 kV-230 kV/RConn1 -- 25km Area 2/LConn1
  25km Area 2/RConn2 -- 10 km Area 2/LConn2 -- T4: 900MVA 20 kV/230 kV/RConn2
  25km Area 2/RConn1 -- 10 km Area 2/LConn1 -- T4: 900MVA 20 kV/230 kV/RConn1
  25km Area 2/RConn3 -- 10 km Area 2/LConn3 -- T4: 900MVA 20 kV/230 kV/RConn3
  10 km Area 2/RConn1 -- 1767MW 100MVAR -187MVAR/LConn1 -- -350MVAR/LConn1 -- A/RConn1
  1767MW 100MVAR -187MVAR/LConn2 -- -350MVAR/LConn2 -- 10 km Area 2/RConn2 -- B/RConn1
  10 km Area 2/RConn3 -- 1767MW 100MVAR -187MVAR/LConn3 -- -350MVAR/LConn3 -- C/RConn1

== system power_kundur_statcom01/Double click here for more info ==

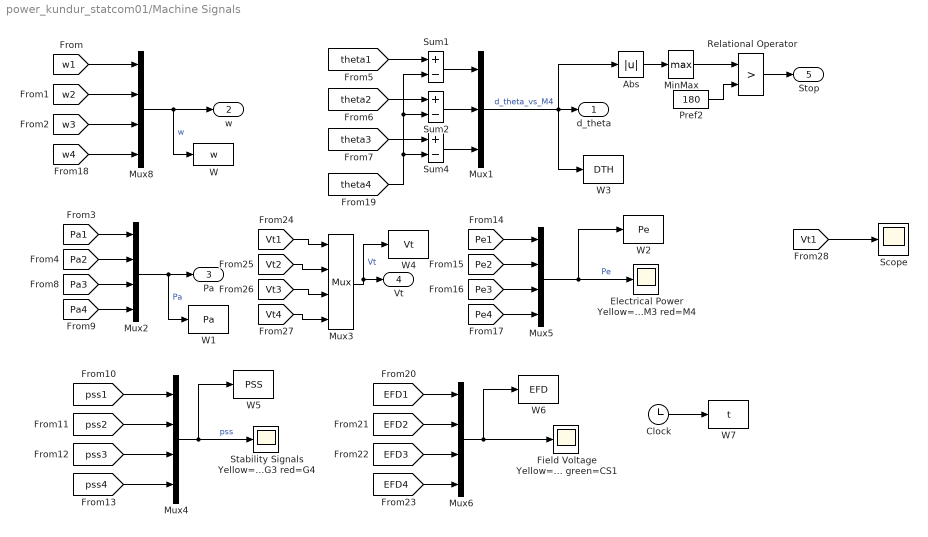
== system power_kundur_statcom01/Machine Signals ==
  Abs : Abs  SaturateOnIntegerOverflow=on
  Clock : Clock
  "Electrical Power Yellow=M1 mag=M2 cyan=M3 red=M4 " : Scope
  Field Voltage Yellow=G1 mag=G2 cyan=G3 red=G4 green=CS1 : Scope
  MinMax : MinMax  Function=max  InputSameDT=on  SaturateOnIntegerOverflow=on
  Mux1 : Mux  Inputs=3
  Mux{2..6,8} (6 alike) : Mux
  Pref2 : Constant  Value=180
  Relational Operator : RelationalOperator  Operator=>  RndMeth=Nearest  InputSameDT=on
  Scope : Scope
  "Stability Signals Yellow=G1 mag=G2 cyan=G3 red=G4 " : Scope
  Sum1 : Sum  Inputs=+-  InputSameDT=on  SaturateOnIntegerOverflow=on  OutDataTypeStr=Inherit: Same as first input
  Sum2 : Sum  Inputs=+-  InputSameDT=on  SaturateOnIntegerOverflow=on  OutDataTypeStr=Inherit: Same as first input
  Sum4 : Sum  Inputs=+-  InputSameDT=on  SaturateOnIntegerOverflow=on  OutDataTypeStr=Inherit: Same as first input
  W : ToWorkspace  VariableName=w  SampleTime=1/60
  W1 : ToWorkspace  VariableName=Pa  SampleTime=1/60
  W2 : ToWorkspace  VariableName=Pe  SampleTime=1/60
  W3 : ToWorkspace  VariableName=DTH  SampleTime=1/60
  W4 : ToWorkspace  VariableName=Vt  SampleTime=1/60
  W5 : ToWorkspace  VariableName=PSS  SampleTime=1/60
  W6 : ToWorkspace  VariableName=EFD  SampleTime=1/60
  W7 : ToWorkspace  VariableName=t  SampleTime=1/60
  d_theta : Outport
  w : Outport  Port=2
  Pa : Outport  Port=3
  Vt : Outport  Port=4
  Stop : Outport  Port=5
  wires:
  Mux1/1 -> d_theta/1, Abs/1, W3/1  "d_theta_vs_M4"
  Abs/1 -> MinMax/1
  Pref2/1 -> Relational Operator/2
  MinMax/1 -> Relational Operator/1
  [Pa1] -> Mux2/1
  Mux4/1 -> "Stability Signals Yellow=G1 mag=G2 cyan=G3 red=G4 "/1, W5/1  "pss"
  [pss1] -> Mux4/1
  [pss2] -> Mux4/2
  [pss4] -> Mux4/4
  [pss3] -> Mux4/3
  [EFD1] -> Mux6/1
  [EFD2] -> Mux6/2
  [EFD4] -> Mux6/4
  [EFD3] -> Mux6/3
  Mux6/1 -> Field Voltage Yellow=G1 mag=G2 cyan=G3 red=G4 green=CS1/1, W6/1
  Mux8/1 -> w/1, W/1  "w"
  Relational Operator/1 -> Stop/1
  Mux2/1 -> Pa/1, W1/1  "Pa"
  [theta1] -> Sum1/1
  Sum1/1 -> Mux1/1
  [theta2] -> Sum2/1
  [theta3] -> Sum4/1
  [theta4] -> Sum4/2, Sum2/2, Sum1/2
  Sum2/1 -> Mux1/2
  Sum4/1 -> Mux1/3
  [Pa2] -> Mux2/2
  [Pa3] -> Mux2/3
  [Pa4] -> Mux2/4
  [Vt1] -> Mux3/1
  [Vt2] -> Mux3/2
  [Vt3] -> Mux3/3
  [Vt4] -> Mux3/4
  Mux3/1 -> Vt/1, W4/1  "Vt"
  [Pe1] -> Mux5/1
  [Pe2] -> Mux5/2
  [Pe3] -> Mux5/3
  [Pe4] -> Mux5/4
  Mux5/1 -> "Electrical Power Yellow=M1 mag=M2 cyan=M3 red=M4 "/1, W2/1  "Pe"
  [w1] -> Mux8/1
  [w2] -> Mux8/2
  [w3] -> Mux8/3
  [w4] -> Mux8/4
  Clock/1 -> W7/1
  [Vt1] -> Scope/1

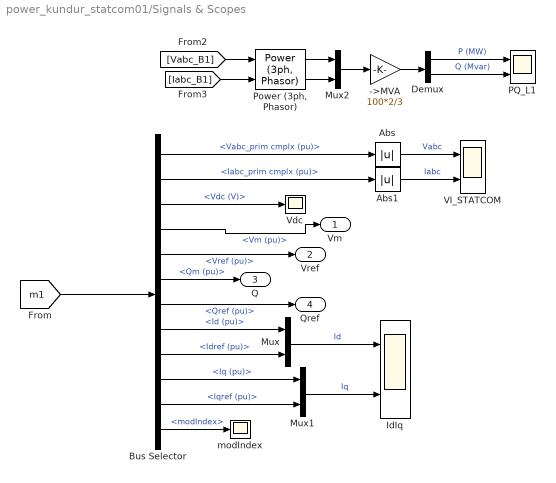
== system power_kundur_statcom01/Signals & Scopes ==
  ->MVA : Gain  Gain=100*2/3
  Abs : Abs
  Abs1 : Abs
  Bus Selector : BusSelector  OutputSignals=Power.Vabc_prim cmplx (pu),Power.Iabc_prim cmplx (pu),Power.Vdc (V),Control.Vm (pu),Control.Vref (pu),Control.Qm (pu),Control.Qref (pu),Control.Id (pu),Control.Idref (pu),Control.Iq (pu),Control.Iqref (pu),Control.modIndex
  Demux : Demux  Outputs=2
  IdIq : Scope  NumInputPorts=2
  Mux : Mux  Inputs=2
  Mux1 : Mux  Inputs=2
  Mux2 : Mux  Inputs=2
  PQ_L1 : Scope  NumInputPorts=2
  "Power (3ph, Phasor)" : spsPower3phPhasorLib/Power (3ph, Phasor)
      settings: SourceProductBaseCode=PS
  VI_STATCOM : Scope  NumInputPorts=2
  Vdc : Scope
  modIndex : Scope
  Vm : Outport
  Vref : Outport  Port=2
  Q : Outport  Port=3
  Qref : Outport  Port=4
  wires:
  Abs/1 -> VI_STATCOM/1  "Vabc"
  Abs1/1 -> VI_STATCOM/2  "Iabc"
  Bus Selector/1 -> Abs/1  "<Vabc_prim cmplx (pu)>"
  Bus Selector/2 -> Abs1/1  "<Iabc_prim cmplx (pu)>"
  Bus Selector/3 -> Vdc/1  "<Vdc (V)>"
  Mux/1 -> IdIq/1  "Id"
  Mux1/1 -> IdIq/2  "Iq"
  Bus Selector/11 -> Mux1/2  "<Iqref (pu)>"
  Bus Selector/12 -> modIndex/1  "<modIndex>"
  Bus Selector/10 -> Mux1/1  "<Iq (pu)>"
  Bus Selector/9 -> Mux/2  "<Idref (pu)>"
  Bus Selector/8 -> Mux/1  "<Id (pu)>"
  Bus Selector/4 -> Vm/1  "<Vm (pu)>"
  Bus Selector/5 -> Vref/1  "<Vref (pu)>"
  Bus Selector/6 -> Q/1  "<Qm (pu)>"
  Bus Selector/7 -> Qref/1  "<Qref (pu)>"
  Demux/1 -> PQ_L1/1  "P (MW)"
  Demux/2 -> PQ_L1/2  "Q (Mvar)"
  ->MVA/1 -> Demux/1
  "Power (3ph, Phasor)"/2 -> Mux2/2
  "Power (3ph, Phasor)"/1 -> Mux2/1
  Mux2/1 -> ->MVA/1
  [Vabc_B1] -> "Power (3ph, Phasor)"/1
  [Iabc_B1] -> "Power (3ph, Phasor)"/2
  [m1] -> Bus Selector/1

== system power_kundur_statcom01/SubSystem ==

== system power_kundur_statcom01/SubSystem3 ==

== system power_kundur_statcom01/SubSystem4 ==

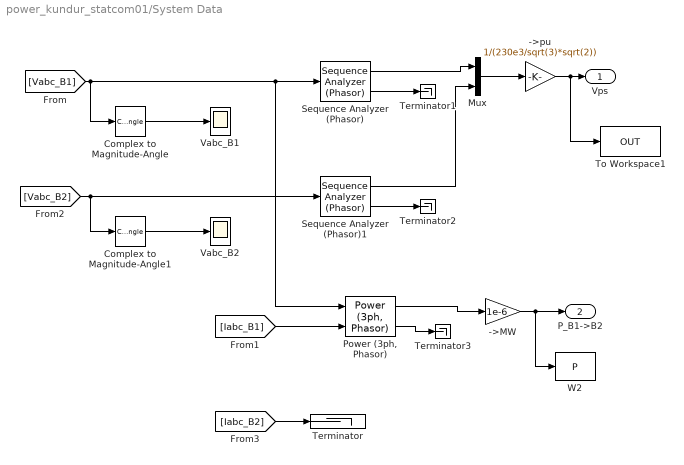
== system power_kundur_statcom01/System Data ==
  ->MW : Gain  Gain=1e-6  SaturateOnIntegerOverflow=on  OutDataTypeStr=Inherit: Same as input  ParamDataTypeStr=Inherit: Same as input
  ->pu : Gain  Gain=1/(230e3/sqrt(3)*sqrt(2))  SaturateOnIntegerOverflow=on  OutDataTypeStr=Inherit: Same as input  ParamDataTypeStr=Inherit: Same as input
  Complex to Magnitude-Angle : ComplexToMagnitudeAngle  Output=Magnitude
  Complex to Magnitude-Angle1 : ComplexToMagnitudeAngle  Output=Magnitude
  Mux : Mux  Inputs=2
  "Power (3ph, Phasor)" : spsPower3phPhasorLib/Power (3ph, Phasor)
      settings: SourceProductBaseCode=PS
  Sequence Analyzer (Phasor) : spsSequenceAnalyzerPhasorLib/Sequence Analyzer (Phasor)  seq=Positive
      settings: SourceProductBaseCode=PS
  Sequence Analyzer (Phasor)1 : spsSequenceAnalyzerPhasorLib/Sequence Analyzer (Phasor)  seq=Positive
      settings: SourceProductBaseCode=PS
  Terminator{,1..3} (4 alike) : Terminator
  To Workspace1 : ToWorkspace  VariableName=OUT  SaveFormat=Timeseries
      settings: Save2DSignal=2-D array (concatenate along first dimension)
  Vabc_B1 : Scope
  Vabc_B2 : Scope
  W2 : ToWorkspace  VariableName=P  SampleTime=1/60
  Vps : Outport
  P_B1->B2 : Outport  Port=2
  wires:
  [Vabc_B1] -> Sequence Analyzer (Phasor)/1, "Power (3ph, Phasor)"/1, Complex to Magnitude-Angle/1
  [Vabc_B2] -> Sequence Analyzer (Phasor)1/1, Complex to Magnitude-Angle1/1
  [Iabc_B2] -> Terminator/1
  Sequence Analyzer (Phasor)/2 -> Terminator1/1
  Sequence Analyzer (Phasor)1/2 -> Terminator2/1
  Sequence Analyzer (Phasor)1/1 -> Mux/2
  [Iabc_B1] -> "Power (3ph, Phasor)"/2
  ->pu/1 -> To Workspace1/1, Vps/1
  Sequence Analyzer (Phasor)/1 -> Mux/1
  Mux/1 -> ->pu/1
  ->MW/1 -> P_B1->B2/1, W2/1
  Complex to Magnitude-Angle/1 -> Vabc_B1/1
  Complex to Magnitude-Angle1/1 -> Vabc_B2/1
  "Power (3ph, Phasor)"/1 -> ->MW/1
  "Power (3ph, Phasor)"/2 -> Terminator3/1

== system power_kundur_statcom01/100 MVA STATCOM1/DC Voltage Computation ==
  Vabc_conv_SH : Inport
  Iabc_SH : Inport  Port=2
  1/C : Gain  Gain=1/C_DC  SaturateOnIntegerOverflow=on  OutDataTypeStr=Inherit: Same as input  ParamDataTypeStr=Inherit: Same as input
  Complex to Real-Imag : ComplexToRealImag
  Gain2 : Gain  Gain=1/2  SaturateOnIntegerOverflow=on  OutDataTypeStr=Inherit: Same as input  ParamDataTypeStr=Inherit: Same as input
  Integrator : Integrator  InitialCondition=VnomDC  LimitOutput=on  UpperSaturationLimit=1000000  LowerSaturationLimit=1e-6
  Math Function1 : Math  Operator=conj  SignedPower=on  SaturateOnIntegerOverflow=on
  Product : Product  SaturateOnIntegerOverflow=on  OutDataTypeStr=Inherit: Same as first input
  Product2 : Product  Inputs=*/  InputSameDT=on  SaturateOnIntegerOverflow=on  OutDataTypeStr=Inherit: Same as first input
  Sum3 : Sum  Inputs=1  InputSameDT=on  SaturateOnIntegerOverflow=on  OutDataTypeStr=Inherit: Same as first input
  Terminator : Terminator
  Vdc : Outport  VectorParamsAs1DForOutWhenUnconnected=off
  wires:
  Gain2/1 -> Complex to Real-Imag/1
  Complex to Real-Imag/1 -> Product2/1  "Pcc=Pca"
  Math Function1/1 -> Product/2
  Vabc_conv_SH/1 -> Product/1
  Sum3/1 -> Gain2/1
  Product/1 -> Sum3/1
  Iabc_SH/1 -> Math Function1/1
  Product2/1 -> 1/C/1  "Idc"
  Integrator/1 -> Product2/2, Vdc/1
  1/C/1 -> Integrator/1
  Complex to Real-Imag/2 -> Terminator/1

== system power_kundur_statcom01/100 MVA STATCOM1/Measurement System ==
  Vabc_prim : Inport  PortDimensions=3  SampleTime=0
  Iabc_prim : Inport  Port=2  PortDimensions=3  SampleTime=0
  "A->pu " : Gain  Gain=Vnom_SH*sqrt(3)/sqrt(2)/Pnom_SH  SaturateOnIntegerOverflow=on  OutDataTypeStr=Inherit: Same as input  ParamDataTypeStr=Inherit: Same as input
  STATCOM Measurement System : Subsystem
  "V->pu " : Gain  Gain=1/(Vnom_SH*sqrt(2)/sqrt(3))  SaturateOnIntegerOverflow=on  OutDataTypeStr=Inherit: Same as input  ParamDataTypeStr=Inherit: Same as input
  Vm : Outport  VectorParamsAs1DForOutWhenUnconnected=off
  Vdq : Outport  Port=2  VectorParamsAs1DForOutWhenUnconnected=off
  Idq : Outport  Port=3  VectorParamsAs1DForOutWhenUnconnected=off
  Qm : Outport  Port=4  VectorParamsAs1DForOutWhenUnconnected=off
  Id_avg : Outport  Port=5  VectorParamsAs1DForOutWhenUnconnected=off
  theta : Outport  Port=6  VectorParamsAs1DForOutWhenUnconnected=off
  wires:
  Vabc_prim/1 -> "V->pu "/1
  Iabc_prim/1 -> "A->pu "/1
  STATCOM Measurement System/1(Vm) -> Vm/1
  STATCOM Measurement System/6(theta) -> theta/1
  STATCOM Measurement System/5(Id_avg) -> Id_avg/1
  "V->pu "/1 -> STATCOM Measurement System/1(Vabc_Prim)
  "A->pu "/1 -> STATCOM Measurement System/2(Iabc_Prim)
  STATCOM Measurement System/2(Vdq) -> Vdq/1
  STATCOM Measurement System/3(Idq) -> Idq/1
  STATCOM Measurement System/4(Qm) -> Qm/1

== system power_kundur_statcom01/100 MVA STATCOM1/Power Components Modeling (Shunt & Series Converter) ==
  Vabc_Conv_SH : Inport  PortDimensions=3
  Trip : Inport  Port=2  PortDimensions=1
  Bus1 : spsThreePhaseVIMeasurementLib/Three-Phase V-I Measurement  VoltageMeasurement=phase-to-ground  SetLabelV=off  LabelV=Vabc_B1x  Vpu=off  VpuLL=off  CurrentMeasurement=yes  SetLabelI=off  LabelI=Iabc_B1x  Ipu=off  Pbase=100e6  Vbase=500e3  OutputType=Complex  PhasorSimulation=on  PSBequivalent=0
  Power Components modeling (Shunt Converter) : Subsystem
  "A1 " : PMIOPort  Side=Left
  B1 : PMIOPort  Port=2  Side=Left
  C1 : PMIOPort  Port=3  Side=Left
  Vabc1 : Outport  VectorParamsAs1DForOutWhenUnconnected=off
  Iabc_SH : Outport  Port=2  VectorParamsAs1DForOutWhenUnconnected=off
  wires:
  [Iabc_prim] -> Iabc_SH/1
  [Vabc_prim] -> Vabc1/1
  [Vabc_prim] -> Power Components modeling (Shunt Converter)/2(Vabc_prim)
  Bus1/2 -> [Iabc_prim]
  Bus1/1 -> [Vabc_prim]
  Vabc_Conv_SH/1 -> Power Components modeling (Shunt Converter)/1(Vabc_Conv)
  Trip/1 -> Power Components modeling (Shunt Converter)/3(Trip_SH)
  connections:
  Power Components modeling (Shunt Converter)/LConn3 -- Bus1/RConn3
  Power Components modeling (Shunt Converter)/LConn2 -- Bus1/RConn2
  Power Components modeling (Shunt Converter)/LConn1 -- Bus1/RConn1
  "A1 "/RConn1 -- Bus1/LConn1
  Bus1/LConn2 -- B1/RConn1
  C1/RConn1 -- Bus1/LConn3

== system power_kundur_statcom01/100 MVA STATCOM1/Shunt Converter Output Voltage Computation ==
  note: V L-L rms = m * sqrt(3)/(2*sqrt(2)) * Vdc
  Vdc : Inport
  m_&_phi : Inport  Port=2
  theta : Inport  Port=3
  A,B,C : Constant  Value=[0 -2*pi/3 2*pi/3]
  Demux : Demux  Outputs=2
      settings: DisplayOption=none
  Kp5 : Gain  Gain=0.5  SaturateOnIntegerOverflow=on  OutDataTypeStr=Inherit: Same as input  ParamDataTypeStr=Inherit: Same as input
  Math Function : Math  SignedPower=on  SaturateOnIntegerOverflow=on
  OpMode : Constant  Value=j
  Product : Product  Inputs=3  SaturateOnIntegerOverflow=on  OutDataTypeStr=Inherit: Same as first input
  Product3 : Product  SaturateOnIntegerOverflow=on  OutDataTypeStr=Inherit: Same as first input
  Sum4 : Sum  Inputs=+++  InputSameDT=on  SaturateOnIntegerOverflow=on  OutDataTypeStr=Inherit: Same as first input
  xfo_ratio_SH : Gain  Gain=xfo_ratio_SH  SaturateOnIntegerOverflow=on  OutDataTypeStr=Inherit: Same as input  ParamDataTypeStr=Inherit: Same as input
  Vabc_Conv : Outport  VectorParamsAs1DForOutWhenUnconnected=off
  wires:
  Math Function/1 -> Product/1
  Product3/1 -> Math Function/1
  OpMode/1 -> Product3/2
  Product/1 -> xfo_ratio_SH/1
  Vdc/1 -> Kp5/1
  A,B,C/1 -> Sum4/1
  Sum4/1 -> Product3/1
  Kp5/1 -> Product/3
  theta/1 -> Sum4/3
  m_&_phi/1 -> Demux/1
  Demux/1 -> Product/2
  Demux/2 -> Sum4/2
  xfo_ratio_SH/1 -> Vabc_Conv/1

== system power_kundur_statcom01/100 MVA STATCOM1/Signals1 ==
  Vabc_prim : Inport
  Iabc_prim : Inport  Port=2
  Vdc : Inport  Port=3
  m_Control : Inport  Port=4
  "A->pu " : Gain  Gain=Vnom_SH*sqrt(3)/sqrt(2)/Pnom_SH  SaturateOnIntegerOverflow=on  OutDataTypeStr=Inherit: Same as input  ParamDataTypeStr=Inherit: Same as input
  Bus Creator : BusCreator  Inputs=9
  Bus Creator1 : BusCreator  Inputs=2
  Bus Creator2 : BusCreator  Inputs=3
  Demux : Demux  Outputs=[1 1 1 1 2 2 1]
      settings: DisplayOption=none
  Demux1 : Demux  Outputs=3
      settings: DisplayOption=none
  Demux2 : Demux  Outputs=3
      settings: DisplayOption=none
  Demux5 : Demux  Outputs=2
      settings: DisplayOption=none
  Demux6 : Demux  Outputs=2
      settings: DisplayOption=none
  Mux : Mux  Inputs=3
  Mux1 : Mux  Inputs=3
  "V->pu " : Gain  Gain=1/(Vnom_SH*sqrt(2)/sqrt(3))  SaturateOnIntegerOverflow=on  OutDataTypeStr=Inherit: Same as input  ParamDataTypeStr=Inherit: Same as input
  m : Outport  VectorParamsAs1DForOutWhenUnconnected=off
  wires:
  "A->pu "/1 -> Demux2/1
  "V->pu "/1 -> Demux1/1
  Vdc/1 -> Bus Creator2/3  "Vdc (V)"
  Demux/2 -> Bus Creator/2  "Vref (pu)"
  Demux/1 -> Bus Creator/1  "Vm (pu)"
  Iabc_prim/1 -> "A->pu "/1
  Bus Creator1/1 -> m/1
  Vabc_prim/1 -> "V->pu "/1
  m_Control/1 -> Demux/1
  Bus Creator2/1 -> Bus Creator1/1  "Power"
  Demux/5 -> Demux5/1
  Demux/6 -> Demux6/1
  Bus Creator/1 -> Bus Creator1/2  "Control"
  Demux/3 -> Bus Creator/3  "Qm (pu)"
  Demux/4 -> Bus Creator/4  "Qref (pu)"
  Demux5/1 -> Bus Creator/5  "Id (pu)"
  Demux5/2 -> Bus Creator/6  "Iq (pu)"
  Demux6/1 -> Bus Creator/7  "Idref (pu)"
  Demux6/2 -> Bus Creator/8  "Iqref (pu)"
  Demux/7 -> Bus Creator/9  "modIndex"
  Demux1/1 -> Mux1/1  "Va_prim (pu)"
  Demux1/2 -> Mux1/2  "Vb_prim (pu)"
  Demux1/3 -> Mux1/3  "Vc_prim (pu)"
  Mux1/1 -> Bus Creator2/1  "Vabc_prim cmplx (pu)"
  Mux/1 -> Bus Creator2/2  "Iabc_prim cmplx (pu)"
  Demux2/1 -> Mux/1  "Ia_prim (pu)"
  Demux2/2 -> Mux/2  "Ib_prim (pu)"
  Demux2/3 -> Mux/3  "Ic_prim (pu)"
